simulink model "SRManCw1_BEZ_MODELU"  (R2018a)
settings: Solver=ode45  StartTime=0.0  StopTime=tend  RelTol=1e-3
model workspace (MAT data in the model file):
  I1 = 0.416666666667
  I2 = 0.16
  L1 = 1
  L2 = 0.8
  Qd1 = 0.1
  Qd2 = 0.2
  b1 = 9.5
  b2 = 4.5
  fC1 = 0.2
  fC2 = 0.1
  g = 9.81
  m1 = 5
  m2 = 3
  tend = 30
  w = 5
settings Model: Creator=szymon  LastModifiedBy=szymon

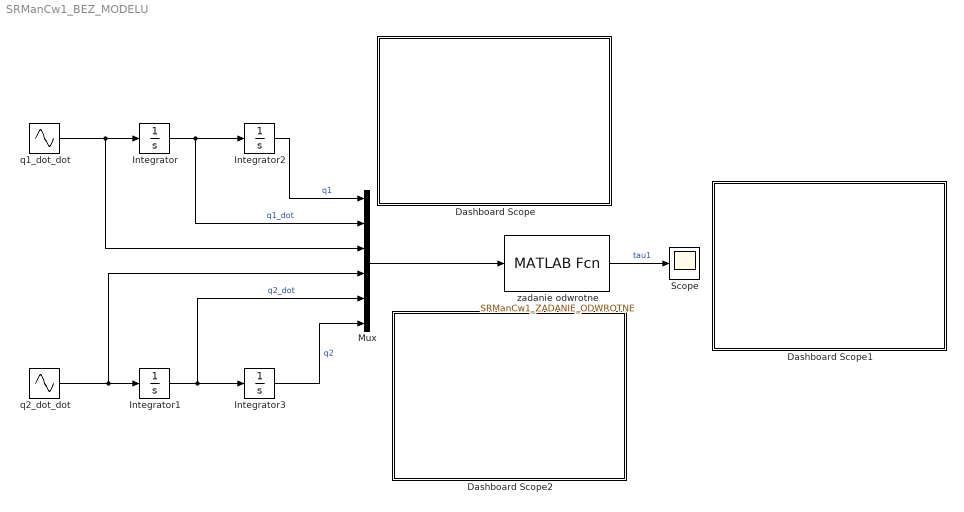
== system SRManCw1_BEZ_MODELU ==
  Dashboard Scope : Subsystem  DialogController=hmiCreateDDGDialog  IsWebBlock=on  mask(MWDashboardBlock){webBlockId=85f042bb-43e3-417a-a2e5-29409c83120d, webBlockType=sdiscope, ShowInitialText=on, HMISrcModelName=SRManCw1_BEZ_MODELU}
      mask prompts: webBlockId "WebBlock Id"; webBlockType "WebBlock Type"; HMISrcModelName "Source Model"
      mask help: SimulinkHMI:dialogs:HMIScopeDialogDesc
      mask Help: helpview([docroot '/mapfiles/simulink.map'], 'hmi_scope')
      mask Display:
      | if strcmp(get_param(bdroot(gcb),'BlockDiagramType'), 'library')
      |     image([(matlabroot) '/toolbox/simulink/hmi/icons/DashboardScope.png']);
      | end
  Dashboard Scope1 : Subsystem  DialogController=hmiCreateDDGDialog  IsWebBlock=on  mask(MWDashboardBlock){webBlockId=cd777eac-a354-456c-9f5d-ab5ff5201cfb, webBlockType=sdiscope, ShowInitialText=on, HMISrcModelName=SRManCw1_BEZ_MODELU}
      mask prompts: webBlockId "WebBlock Id"; webBlockType "WebBlock Type"; HMISrcModelName "Source Model"
      mask help: SimulinkHMI:dialogs:HMIScopeDialogDesc
      mask Help: helpview([docroot '/mapfiles/simulink.map'], 'hmi_scope')
      mask Display:
      | if strcmp(get_param(bdroot(gcb),'BlockDiagramType'), 'library')
      |     image([(matlabroot) '/toolbox/simulink/hmi/icons/DashboardScope.png']);
      | end
  Dashboard Scope2 : Subsystem  DialogController=hmiCreateDDGDialog  IsWebBlock=on  mask(MWDashboardBlock){webBlockId=b849867b-a4a0-4224-a1ea-8274c603c54b, webBlockType=sdiscope, ShowInitialText=on, HMISrcModelName=SRManCw1_BEZ_MODELU}
      mask prompts: webBlockId "WebBlock Id"; webBlockType "WebBlock Type"; HMISrcModelName "Source Model"
      mask help: SimulinkHMI:dialogs:HMIScopeDialogDesc
      mask Help: helpview([docroot '/mapfiles/simulink.map'], 'hmi_scope')
      mask Display:
      | if strcmp(get_param(bdroot(gcb),'BlockDiagramType'), 'library')
      |     image([(matlabroot) '/toolbox/simulink/hmi/icons/DashboardScope.png']);
      | end
  Integrator{,1..3} (4 alike) : Integrator
  Mux : Mux  Inputs=6
  Scope : Scope
  "q1_dot_dot " : Sin  Amplitude=-w^2*Qd1  SampleTime=0
  "q2_dot_dot " : Sin  Amplitude=-w^2*Qd2  SampleTime=0
  zadanie odwrotne : MATLABFcn  MATLABFcn=SRManCw1_ZADANIE_ODWROTNE
  wires:
  Mux/1 -> zadanie odwrotne/1
  "q1_dot_dot "/1 -> Mux/3, Integrator/1
  Integrator/1 -> Mux/2, Integrator2/1  "q1_dot"
  "q2_dot_dot "/1 -> Mux/4, Integrator1/1
  Integrator1/1 -> Mux/5, Integrator3/1  "q2_dot"
  Integrator2/1 -> Mux/1  "q1"
  Integrator3/1 -> Mux/6  "q2"
  zadanie odwrotne/1 -> Scope/1  "tau1"

== system SRManCw1_BEZ_MODELU/Dashboard Scope ==

== system SRManCw1_BEZ_MODELU/Dashboard Scope1 ==

== system SRManCw1_BEZ_MODELU/Dashboard Scope2 ==
